simulink model "DpfIntfc_Delivery"  (Simulink 8.2)
settings: Solver=FixedStepDiscrete  StartTime=0.0  StopTime=10.0  FixedStep=0.001  RelTol=1e-3
undefined symbols (not defined in the file): DiscIntNeverNeededParam
libraries: simulink x15, DpfIntfc_Lib x1
(part 1 of 2)
settings Model: Creator=u13x50  LastModifiedBy=u13x50
settings DataIOCC: LimitDataPoints=off  SignalLoggingSaveFormat=Dataset  SaveOutput=off  SaveTime=off
settings OptimizationCC: InlineParams=on  ZeroExternalMemoryAtStartup=off  ZeroInternalMemoryAtStartup=off  InitFltsAndDblsToZero=on  EfficientMapNaN2IntZero=off  OptimizeModelRefInitCode=on  LifeSpan=Inf
settings DebuggingCC: SignalInfNanChecking=error  SignalRangeChecking=error  ReadBeforeWriteMsg=DisableAll  WriteAfterWriteMsg=DisableAll  WriteAfterReadMsg=DisableAll  InheritedTsInSrcMsg=none  UnderSpecifiedDataTypeMsg=error
settings ModelReferenceCC: ModelReferenceNumInstancesAllowed=Single
settings RTWCC: SystemTargetFile=ert.tlc  GenCodeOnly=on  GenerateMakefile=off  TemplateMakefile=ert_default_tmf  Description=Embedded Coder  GenerateReport=on  ProcessScript=ert_make_rtw_hook  IncludeHyperlinkInReport=on  LaunchReport=on
settings CodeAppCC: IgnoreCustomStorageClasses=off  CustomSymbolStrType=$N$R$M  SimulinkBlockComments=off  InternalIdentifier=Classic
settings ERTTargetCC: CodeReplacementLibrary=ANSI_C  UtilityFuncGeneration=Shared location  MultiwordLength=2048  IncludeMdlTerminateFcn=off  SuppressErrorStatus=on  SupportNonFinite=off  SupportComplex=off  ParenthesesLevel=Maximum  InlinedParameterPlacement=NonHierarchical  ERTCustomFileTemplate=example_file_process.tlc  ConvertIfToSwitch=off  SuppressUnreachableDefaultCases=off

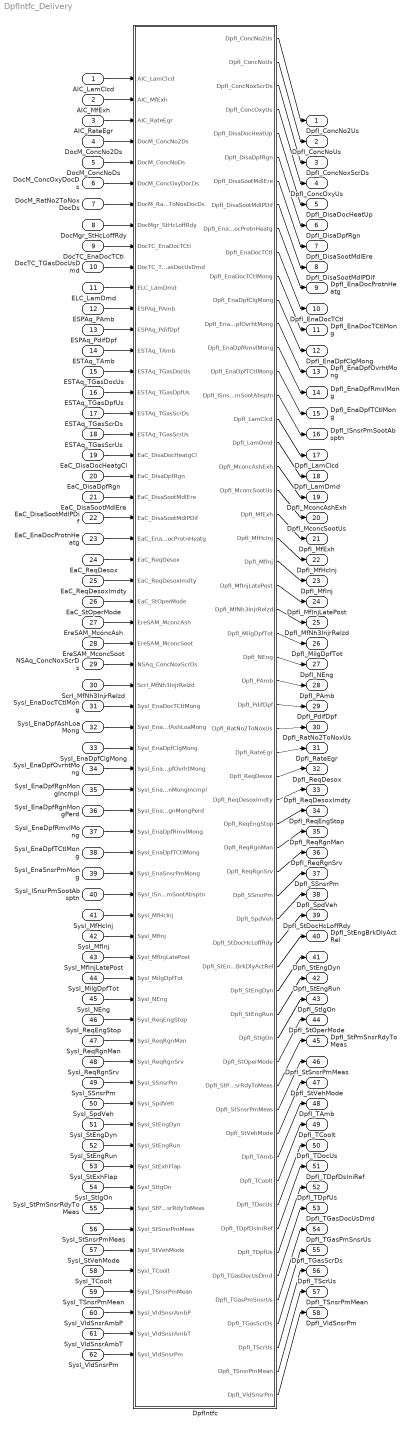
== system DpfIntfc_Delivery ==
  AIC_LamClcd : Inport
  AIC_MfExh : Inport  Port=2
  AIC_RateEgr : Inport  Port=3
  DocM_ConcNo2Ds : Inport  Port=4
  DocM_ConcNoDs : Inport  Port=5
  DocM_ConcOxyDocDs : Inport  Port=6
  DocM_RatNo2ToNoxDocDs : Inport  Port=7
  DocMgr_StHcLoffRdy : Inport  Port=8
  DocTC_EnaDocTCtl : Inport  Port=9
  DocTC_TGasDocUsDmd : Inport  Port=10
  ELC_LamDmd : Inport  Port=11
  ESPAq_PAmb : Inport  Port=12
  ESPAq_PdifDpf : Inport  Port=13
  ESTAq_TAmb : Inport  Port=14
  ESTAq_TGasDocUs : Inport  Port=15
  ESTAq_TGasDpfUs : Inport  Port=16
  ESTAq_TGasScrDs : Inport  Port=17
  ESTAq_TGasScrUs : Inport  Port=18
  EaC_DisaDocHeatgCl : Inport  Port=19
  EaC_DisaDpfRgn : Inport  Port=20
  EaC_DisaSootMdlEre : Inport  Port=21
  EaC_DisaSootMdlPDif : Inport  Port=22
  EaC_EnaDocProtnHeatg : Inport  Port=23
  EaC_ReqDesox : Inport  Port=24
  EaC_ReqDesoxImdty : Inport  Port=25
  EaC_StOperMode : Inport  Port=26
  EreSAM_MconcAsh : Inport  Port=27
  EreSAM_MconcSoot : Inport  Port=28
  NSAq_ConcNoxScrDs : Inport  Port=29
  ScrI_MfNh3InjrRelzd : Inport  Port=30
  SysI_EnaDocTCtlMong : Inport  Port=31
  SysI_EnaDpfAshLoaMong : Inport  Port=32
  SysI_EnaDpfClgMong : Inport  Port=33
  SysI_EnaDpfOvrhtMong : Inport  Port=34
  SysI_EnaDpfRgnMongIncmpl : Inport  Port=35
  SysI_EnaDpfRgnMongPerd : Inport  Port=36
  SysI_EnaDpfRmvlMong : Inport  Port=37
  SysI_EnaDpfTCtlMong : Inport  Port=38
  SysI_EnaSnsrPmMong : Inport  Port=39
  SysI_ISnsrPmSootAbsptn : Inport  Port=40
  SysI_MfHcInj : Inport  Port=41
  SysI_MfInj : Inport  Port=42
  SysI_MfInjLatePost : Inport  Port=43
  SysI_MilgDpfTot : Inport  Port=44
  SysI_NEng : Inport  Port=45
  SysI_ReqEngStop : Inport  Port=46
  SysI_ReqRgnMan : Inport  Port=47
  SysI_ReqRgnSrv : Inport  Port=48
  SysI_SSnsrPm : Inport  Port=49
  SysI_SpdVeh : Inport  Port=50
  SysI_StEngDyn : Inport  Port=51
  SysI_StEngRun : Inport  Port=52
  SysI_StExhFlap : Inport  Port=53
  SysI_StIgOn : Inport  Port=54
  SysI_StPmSnsrRdyToMeas : Inport  Port=55
  SysI_StSnsrPmMeas : Inport  Port=56
  SysI_StVehMode : Inport  Port=57
  SysI_TCoolt : Inport  Port=58
  SysI_TSnsrPmMean : Inport  Port=59
  SysI_VldSnsrAmbP : Inport  Port=60
  SysI_VldSnsrAmbT : Inport  Port=61
  SysI_VldSnsrPm : Inport  Port=62
  DpfIntfc : Subsystem
  DpfI_ConcNo2Us : Outport
  DpfI_ConcNoUs : Outport  Port=2
  DpfI_ConcNoxScrDs : Outport  Port=3
  DpfI_ConcOxyUs : Outport  Port=4
  DpfI_DisaDocHeatUp : Outport  Port=5
  DpfI_DisaDpfRgn : Outport  Port=6
  DpfI_DisaSootMdlEre : Outport  Port=7
  DpfI_DisaSootMdlPDif : Outport  Port=8
  DpfI_EnaDocProtnHeatg : Outport  Port=9
  DpfI_EnaDocTCtl : Outport  Port=10
  DpfI_EnaDocTCtlMong : Outport  Port=11
  DpfI_EnaDpfClgMong : Outport  Port=12
  DpfI_EnaDpfOvrhtMong : Outport  Port=13
  DpfI_EnaDpfRmvlMong : Outport  Port=14
  DpfI_EnaDpfTCtlMong : Outport  Port=15
  DpfI_ISnsrPmSootAbsptn : Outport  Port=16
  DpfI_LamClcd : Outport  Port=17
  DpfI_LamDmd : Outport  Port=18
  DpfI_MconcAshExh : Outport  Port=19
  DpfI_MconcSootUs : Outport  Port=20
  DpfI_MfExh : Outport  Port=21
  DpfI_MfHcInj : Outport  Port=22
  DpfI_MfInj : Outport  Port=23
  DpfI_MfInjLatePost : Outport  Port=24
  DpfI_MfNh3InjrRelzd : Outport  Port=25
  DpfI_MilgDpfTot : Outport  Port=26
  DpfI_NEng : Outport  Port=27
  DpfI_PAmb : Outport  Port=28
  DpfI_PdifDpf : Outport  Port=29
  DpfI_RatNo2ToNoxUs : Outport  Port=30
  DpfI_RateEgr : Outport  Port=31
  DpfI_ReqDesox : Outport  Port=32
  DpfI_ReqDesoxImdty : Outport  Port=33
  DpfI_ReqEngStop : Outport  Port=34
  DpfI_ReqRgnMan : Outport  Port=35
  DpfI_ReqRgnSrv : Outport  Port=36
  DpfI_SSnsrPm : Outport  Port=37
  DpfI_SpdVeh : Outport  Port=38
  DpfI_StDocHcLoffRdy : Outport  Port=39
  DpfI_StEngBrkDlyActRel : Outport  Port=40
  DpfI_StEngDyn : Outport  Port=41
  DpfI_StEngRun : Outport  Port=42
  DpfI_StIgOn : Outport  Port=43
  DpfI_StOperMode : Outport  Port=44
  DpfI_StPmSnsrRdyToMeas : Outport  Port=45
  DpfI_StSnsrPmMeas : Outport  Port=46
  DpfI_StVehMode : Outport  Port=47
  DpfI_TAmb : Outport  Port=48
  DpfI_TCoolt : Outport  Port=49
  DpfI_TDocUs : Outport  Port=50
  DpfI_TDpfDsIniRef : Outport  Port=51
  DpfI_TDpfUs : Outport  Port=52
  DpfI_TGasDocUsDmd : Outport  Port=53
  DpfI_TGasPmSnsrUs : Outport  Port=54
  DpfI_TGasScrDs : Outport  Port=55
  DpfI_TScrUs : Outport  Port=56
  DpfI_TSnsrPmMean : Outport  Port=57
  DpfI_VldSnsrPm : Outport  Port=58
  wires:
  AIC_LamClcd/1 -> DpfIntfc/1(AIC_LamClcd)
  AIC_MfExh/1 -> DpfIntfc/2(AIC_MfExh)
  AIC_RateEgr/1 -> DpfIntfc/3(AIC_RateEgr)
  DocM_ConcNo2Ds/1 -> DpfIntfc/4(DocM_ConcNo2Ds)
  DocM_ConcNoDs/1 -> DpfIntfc/5(DocM_ConcNoDs)
  DocM_ConcOxyDocDs/1 -> DpfIntfc/6(DocM_ConcOxyDocDs)
  DocM_RatNo2ToNoxDocDs/1 -> DpfIntfc/7(DocM_RatNo2ToNoxDocDs)
  DocMgr_StHcLoffRdy/1 -> DpfIntfc/8(DocMgr_StHcLoffRdy)
  DocTC_EnaDocTCtl/1 -> DpfIntfc/9(DocTC_EnaDocTCtl)
  DocTC_TGasDocUsDmd/1 -> DpfIntfc/10(DocTC_TGasDocUsDmd)
  ELC_LamDmd/1 -> DpfIntfc/11(ELC_LamDmd)
  ESPAq_PAmb/1 -> DpfIntfc/12(ESPAq_PAmb)
  ESPAq_PdifDpf/1 -> DpfIntfc/13(ESPAq_PdifDpf)
  ESTAq_TAmb/1 -> DpfIntfc/14(ESTAq_TAmb)
  ESTAq_TGasDocUs/1 -> DpfIntfc/15(ESTAq_TGasDocUs)
  ESTAq_TGasDpfUs/1 -> DpfIntfc/16(ESTAq_TGasDpfUs)
  ESTAq_TGasScrDs/1 -> DpfIntfc/17(ESTAq_TGasScrDs)
  ESTAq_TGasScrUs/1 -> DpfIntfc/18(ESTAq_TGasScrUs)
  EaC_DisaDocHeatgCl/1 -> DpfIntfc/19(EaC_DisaDocHeatgCl)
  EaC_DisaDpfRgn/1 -> DpfIntfc/20(EaC_DisaDpfRgn)
  EaC_DisaSootMdlEre/1 -> DpfIntfc/21(EaC_DisaSootMdlEre)
  EaC_DisaSootMdlPDif/1 -> DpfIntfc/22(EaC_DisaSootMdlPDif)
  EaC_EnaDocProtnHeatg/1 -> DpfIntfc/23(EaC_EnaDocProtnHeatg)
  EaC_ReqDesox/1 -> DpfIntfc/24(EaC_ReqDesox)
  EaC_ReqDesoxImdty/1 -> DpfIntfc/25(EaC_ReqDesoxImdty)
  EaC_StOperMode/1 -> DpfIntfc/26(EaC_StOperMode)
  EreSAM_MconcAsh/1 -> DpfIntfc/27(EreSAM_MconcAsh)
  EreSAM_MconcSoot/1 -> DpfIntfc/28(EreSAM_MconcSoot)
  NSAq_ConcNoxScrDs/1 -> DpfIntfc/29(NSAq_ConcNoxScrDs)
  ScrI_MfNh3InjrRelzd/1 -> DpfIntfc/30(ScrI_MfNh3InjrRelzd)
  SysI_EnaDocTCtlMong/1 -> DpfIntfc/31(SysI_EnaDocTCtlMong)
  SysI_EnaDpfAshLoaMong/1 -> DpfIntfc/32(SysI_EnaDpfAshLoaMong)
  SysI_EnaDpfClgMong/1 -> DpfIntfc/33(SysI_EnaDpfClgMong)
  SysI_EnaDpfOvrhtMong/1 -> DpfIntfc/34(SysI_EnaDpfOvrhtMong)
  SysI_EnaDpfRgnMongIncmpl/1 -> DpfIntfc/35(SysI_EnaDpfRgnMongIncmpl)
  SysI_EnaDpfRgnMongPerd/1 -> DpfIntfc/36(SysI_EnaDpfRgnMongPerd)
  SysI_EnaDpfRmvlMong/1 -> DpfIntfc/37(SysI_EnaDpfRmvlMong)
  SysI_EnaDpfTCtlMong/1 -> DpfIntfc/38(SysI_EnaDpfTCtlMong)
  SysI_EnaSnsrPmMong/1 -> DpfIntfc/39(SysI_EnaSnsrPmMong)
  SysI_ISnsrPmSootAbsptn/1 -> DpfIntfc/40(SysI_ISnsrPmSootAbsptn)
  SysI_MfHcInj/1 -> DpfIntfc/41(SysI_MfHcInj)
  SysI_MfInj/1 -> DpfIntfc/42(SysI_MfInj)
  SysI_MfInjLatePost/1 -> DpfIntfc/43(SysI_MfInjLatePost)
  SysI_MilgDpfTot/1 -> DpfIntfc/44(SysI_MilgDpfTot)
  SysI_NEng/1 -> DpfIntfc/45(SysI_NEng)
  SysI_ReqEngStop/1 -> DpfIntfc/46(SysI_ReqEngStop)
  SysI_ReqRgnMan/1 -> DpfIntfc/47(SysI_ReqRgnMan)
  SysI_ReqRgnSrv/1 -> DpfIntfc/48(SysI_ReqRgnSrv)
  SysI_SSnsrPm/1 -> DpfIntfc/49(SysI_SSnsrPm)
  SysI_SpdVeh/1 -> DpfIntfc/50(SysI_SpdVeh)
  SysI_StEngDyn/1 -> DpfIntfc/51(SysI_StEngDyn)
  SysI_StEngRun/1 -> DpfIntfc/52(SysI_StEngRun)
  SysI_StExhFlap/1 -> DpfIntfc/53(SysI_StExhFlap)
  SysI_StIgOn/1 -> DpfIntfc/54(SysI_StIgOn)
  SysI_StPmSnsrRdyToMeas/1 -> DpfIntfc/55(SysI_StPmSnsrRdyToMeas)
  SysI_StSnsrPmMeas/1 -> DpfIntfc/56(SysI_StSnsrPmMeas)
  SysI_StVehMode/1 -> DpfIntfc/57(SysI_StVehMode)
  SysI_TCoolt/1 -> DpfIntfc/58(SysI_TCoolt)
  SysI_TSnsrPmMean/1 -> DpfIntfc/59(SysI_TSnsrPmMean)
  SysI_VldSnsrAmbP/1 -> DpfIntfc/60(SysI_VldSnsrAmbP)
  SysI_VldSnsrAmbT/1 -> DpfIntfc/61(SysI_VldSnsrAmbT)
  SysI_VldSnsrPm/1 -> DpfIntfc/62(SysI_VldSnsrPm)
  DpfIntfc/1(DpfI_ConcNo2Us) -> DpfI_ConcNo2Us/1
  DpfIntfc/2(DpfI_ConcNoUs) -> DpfI_ConcNoUs/1
  DpfIntfc/3(DpfI_ConcNoxScrDs) -> DpfI_ConcNoxScrDs/1
  DpfIntfc/4(DpfI_ConcOxyUs) -> DpfI_ConcOxyUs/1
  DpfIntfc/5(DpfI_DisaDocHeatUp) -> DpfI_DisaDocHeatUp/1
  DpfIntfc/6(DpfI_DisaDpfRgn) -> DpfI_DisaDpfRgn/1
  DpfIntfc/7(DpfI_DisaSootMdlEre) -> DpfI_DisaSootMdlEre/1
  DpfIntfc/8(DpfI_DisaSootMdlPDif) -> DpfI_DisaSootMdlPDif/1
  DpfIntfc/9(DpfI_EnaDocProtnHeatg) -> DpfI_EnaDocProtnHeatg/1
  DpfIntfc/10(DpfI_EnaDocTCtl) -> DpfI_EnaDocTCtl/1
  DpfIntfc/11(DpfI_EnaDocTCtlMong) -> DpfI_EnaDocTCtlMong/1
  DpfIntfc/12(DpfI_EnaDpfClgMong) -> DpfI_EnaDpfClgMong/1
  DpfIntfc/13(DpfI_EnaDpfOvrhtMong) -> DpfI_EnaDpfOvrhtMong/1
  DpfIntfc/14(DpfI_EnaDpfRmvlMong) -> DpfI_EnaDpfRmvlMong/1
  DpfIntfc/15(DpfI_EnaDpfTCtlMong) -> DpfI_EnaDpfTCtlMong/1
  DpfIntfc/16(DpfI_ISnsrPmSootAbsptn) -> DpfI_ISnsrPmSootAbsptn/1
  DpfIntfc/17(DpfI_LamClcd) -> DpfI_LamClcd/1
  DpfIntfc/18(DpfI_LamDmd) -> DpfI_LamDmd/1
  DpfIntfc/19(DpfI_MconcAshExh) -> DpfI_MconcAshExh/1
  DpfIntfc/20(DpfI_MconcSootUs) -> DpfI_MconcSootUs/1
  DpfIntfc/21(DpfI_MfExh) -> DpfI_MfExh/1
  DpfIntfc/22(DpfI_MfHcInj) -> DpfI_MfHcInj/1
  DpfIntfc/23(DpfI_MfInj) -> DpfI_MfInj/1
  DpfIntfc/24(DpfI_MfInjLatePost) -> DpfI_MfInjLatePost/1
  DpfIntfc/25(DpfI_MfNh3InjrRelzd) -> DpfI_MfNh3InjrRelzd/1
  DpfIntfc/26(DpfI_MilgDpfTot) -> DpfI_MilgDpfTot/1
  DpfIntfc/27(DpfI_NEng) -> DpfI_NEng/1
  DpfIntfc/28(DpfI_PAmb) -> DpfI_PAmb/1
  DpfIntfc/29(DpfI_PdifDpf) -> DpfI_PdifDpf/1
  DpfIntfc/30(DpfI_RatNo2ToNoxUs) -> DpfI_RatNo2ToNoxUs/1
  DpfIntfc/31(DpfI_RateEgr) -> DpfI_RateEgr/1
  DpfIntfc/32(DpfI_ReqDesox) -> DpfI_ReqDesox/1
  DpfIntfc/33(DpfI_ReqDesoxImdty) -> DpfI_ReqDesoxImdty/1
  DpfIntfc/34(DpfI_ReqEngStop) -> DpfI_ReqEngStop/1
  DpfIntfc/35(DpfI_ReqRgnMan) -> DpfI_ReqRgnMan/1
  DpfIntfc/36(DpfI_ReqRgnSrv) -> DpfI_ReqRgnSrv/1
  DpfIntfc/37(DpfI_SSnsrPm) -> DpfI_SSnsrPm/1
  DpfIntfc/38(DpfI_SpdVeh) -> DpfI_SpdVeh/1
  DpfIntfc/39(DpfI_StDocHcLoffRdy) -> DpfI_StDocHcLoffRdy/1
  DpfIntfc/40(DpfI_StEngBrkDlyActRel) -> DpfI_StEngBrkDlyActRel/1
  DpfIntfc/41(DpfI_StEngDyn) -> DpfI_StEngDyn/1
  DpfIntfc/42(DpfI_StEngRun) -> DpfI_StEngRun/1
  DpfIntfc/43(DpfI_StIgOn) -> DpfI_StIgOn/1
  DpfIntfc/44(DpfI_StOperMode) -> DpfI_StOperMode/1
  DpfIntfc/45(DpfI_StPmSnsrRdyToMeas) -> DpfI_StPmSnsrRdyToMeas/1
  DpfIntfc/46(DpfI_StSnsrPmMeas) -> DpfI_StSnsrPmMeas/1
  DpfIntfc/47(DpfI_StVehMode) -> DpfI_StVehMode/1
  DpfIntfc/48(DpfI_TAmb) -> DpfI_TAmb/1
  DpfIntfc/49(DpfI_TCoolt) -> DpfI_TCoolt/1
  DpfIntfc/50(DpfI_TDocUs) -> DpfI_TDocUs/1
  DpfIntfc/51(DpfI_TDpfDsIniRef) -> DpfI_TDpfDsIniRef/1
  DpfIntfc/52(DpfI_TDpfUs) -> DpfI_TDpfUs/1
  DpfIntfc/53(DpfI_TGasDocUsDmd) -> DpfI_TGasDocUsDmd/1
  DpfIntfc/54(DpfI_TGasPmSnsrUs) -> DpfI_TGasPmSnsrUs/1
  DpfIntfc/55(DpfI_TGasScrDs) -> DpfI_TGasScrDs/1
  DpfIntfc/56(DpfI_TScrUs) -> DpfI_TScrUs/1
  DpfIntfc/57(DpfI_TSnsrPmMean) -> DpfI_TSnsrPmMean/1
  DpfIntfc/58(DpfI_VldSnsrPm) -> DpfI_VldSnsrPm/1

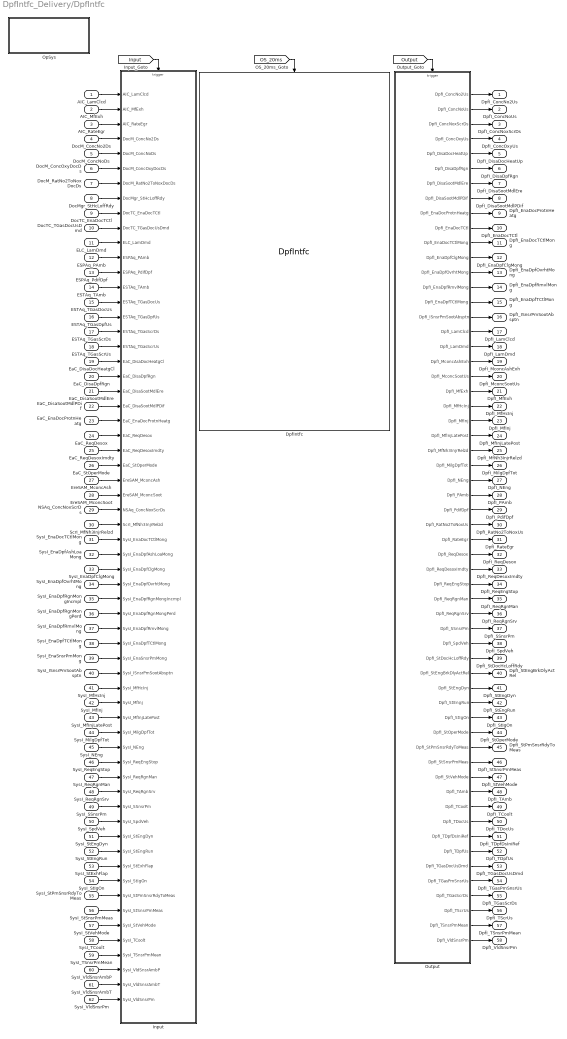
== system DpfIntfc_Delivery/DpfIntfc ==
  AIC_LamClcd : Inport
  AIC_MfExh : Inport  Port=2
  AIC_RateEgr : Inport  Port=3
  DocM_ConcNo2Ds : Inport  Port=4
  DocM_ConcNoDs : Inport  Port=5
  DocM_ConcOxyDocDs : Inport  Port=6
  DocM_RatNo2ToNoxDocDs : Inport  Port=7
  DocMgr_StHcLoffRdy : Inport  Port=8
  DocTC_EnaDocTCtl : Inport  Port=9
  DocTC_TGasDocUsDmd : Inport  Port=10
  ELC_LamDmd : Inport  Port=11
  ESPAq_PAmb : Inport  Port=12
  ESPAq_PdifDpf : Inport  Port=13
  ESTAq_TAmb : Inport  Port=14
  ESTAq_TGasDocUs : Inport  Port=15
  ESTAq_TGasDpfUs : Inport  Port=16
  ESTAq_TGasScrDs : Inport  Port=17
  ESTAq_TGasScrUs : Inport  Port=18
  EaC_DisaDocHeatgCl : Inport  Port=19
  EaC_DisaDpfRgn : Inport  Port=20
  EaC_DisaSootMdlEre : Inport  Port=21
  EaC_DisaSootMdlPDif : Inport  Port=22
  EaC_EnaDocProtnHeatg : Inport  Port=23
  EaC_ReqDesox : Inport  Port=24
  EaC_ReqDesoxImdty : Inport  Port=25
  EaC_StOperMode : Inport  Port=26
  EreSAM_MconcAsh : Inport  Port=27
  EreSAM_MconcSoot : Inport  Port=28
  NSAq_ConcNoxScrDs : Inport  Port=29
  ScrI_MfNh3InjrRelzd : Inport  Port=30
  SysI_EnaDocTCtlMong : Inport  Port=31
  SysI_EnaDpfAshLoaMong : Inport  Port=32
  SysI_EnaDpfClgMong : Inport  Port=33
  SysI_EnaDpfOvrhtMong : Inport  Port=34
  SysI_EnaDpfRgnMongIncmpl : Inport  Port=35
  SysI_EnaDpfRgnMongPerd : Inport  Port=36
  SysI_EnaDpfRmvlMong : Inport  Port=37
  SysI_EnaDpfTCtlMong : Inport  Port=38
  SysI_EnaSnsrPmMong : Inport  Port=39
  SysI_ISnsrPmSootAbsptn : Inport  Port=40
  SysI_MfHcInj : Inport  Port=41
  SysI_MfInj : Inport  Port=42
  SysI_MfInjLatePost : Inport  Port=43
  SysI_MilgDpfTot : Inport  Port=44
  SysI_NEng : Inport  Port=45
  SysI_ReqEngStop : Inport  Port=46
  SysI_ReqRgnMan : Inport  Port=47
  SysI_ReqRgnSrv : Inport  Port=48
  SysI_SSnsrPm : Inport  Port=49
  SysI_SpdVeh : Inport  Port=50
  SysI_StEngDyn : Inport  Port=51
  SysI_StEngRun : Inport  Port=52
  SysI_StExhFlap : Inport  Port=53
  SysI_StIgOn : Inport  Port=54
  SysI_StPmSnsrRdyToMeas : Inport  Port=55
  SysI_StSnsrPmMeas : Inport  Port=56
  SysI_StVehMode : Inport  Port=57
  SysI_TCoolt : Inport  Port=58
  SysI_TSnsrPmMean : Inport  Port=59
  SysI_VldSnsrAmbP : Inport  Port=60
  SysI_VldSnsrAmbT : Inport  Port=61
  SysI_VldSnsrPm : Inport  Port=62
  DpfIntfc : DpfIntfc_Lib/DpfIntfc  SystemSampleTime=-1
  Input : Subsystem  TreatAsAtomicUnit=on
  OpSys : Subsystem
      mask Display: disp('Operating System')
  Output : Subsystem  TreatAsAtomicUnit=on
  DpfI_ConcNo2Us : Outport
  DpfI_ConcNoUs : Outport  Port=2
  DpfI_ConcNoxScrDs : Outport  Port=3
  DpfI_ConcOxyUs : Outport  Port=4
  DpfI_DisaDocHeatUp : Outport  Port=5
  DpfI_DisaDpfRgn : Outport  Port=6
  DpfI_DisaSootMdlEre : Outport  Port=7
  DpfI_DisaSootMdlPDif : Outport  Port=8
  DpfI_EnaDocProtnHeatg : Outport  Port=9
  DpfI_EnaDocTCtl : Outport  Port=10
  DpfI_EnaDocTCtlMong : Outport  Port=11
  DpfI_EnaDpfClgMong : Outport  Port=12
  DpfI_EnaDpfOvrhtMong : Outport  Port=13
  DpfI_EnaDpfRmvlMong : Outport  Port=14
  DpfI_EnaDpfTCtlMong : Outport  Port=15
  DpfI_ISnsrPmSootAbsptn : Outport  Port=16
  DpfI_LamClcd : Outport  Port=17
  DpfI_LamDmd : Outport  Port=18
  DpfI_MconcAshExh : Outport  Port=19
  DpfI_MconcSootUs : Outport  Port=20
  DpfI_MfExh : Outport  Port=21
  DpfI_MfHcInj : Outport  Port=22
  DpfI_MfInj : Outport  Port=23
  DpfI_MfInjLatePost : Outport  Port=24
  DpfI_MfNh3InjrRelzd : Outport  Port=25
  DpfI_MilgDpfTot : Outport  Port=26
  DpfI_NEng : Outport  Port=27
  DpfI_PAmb : Outport  Port=28
  DpfI_PdifDpf : Outport  Port=29
  DpfI_RatNo2ToNoxUs : Outport  Port=30
  DpfI_RateEgr : Outport  Port=31
  DpfI_ReqDesox : Outport  Port=32
  DpfI_ReqDesoxImdty : Outport  Port=33
  DpfI_ReqEngStop : Outport  Port=34
  DpfI_ReqRgnMan : Outport  Port=35
  DpfI_ReqRgnSrv : Outport  Port=36
  DpfI_SSnsrPm : Outport  Port=37
  DpfI_SpdVeh : Outport  Port=38
  DpfI_StDocHcLoffRdy : Outport  Port=39
  DpfI_StEngBrkDlyActRel : Outport  Port=40
  DpfI_StEngDyn : Outport  Port=41
  DpfI_StEngRun : Outport  Port=42
  DpfI_StIgOn : Outport  Port=43
  DpfI_StOperMode : Outport  Port=44
  DpfI_StPmSnsrRdyToMeas : Outport  Port=45
  DpfI_StSnsrPmMeas : Outport  Port=46
  DpfI_StVehMode : Outport  Port=47
  DpfI_TAmb : Outport  Port=48
  DpfI_TCoolt : Outport  Port=49
  DpfI_TDocUs : Outport  Port=50
  DpfI_TDpfDsIniRef : Outport  Port=51
  DpfI_TDpfUs : Outport  Port=52
  DpfI_TGasDocUsDmd : Outport  Port=53
  DpfI_TGasPmSnsrUs : Outport  Port=54
  DpfI_TGasScrDs : Outport  Port=55
  DpfI_TScrUs : Outport  Port=56
  DpfI_TSnsrPmMean : Outport  Port=57
  DpfI_VldSnsrPm : Outport  Port=58
  wires:
  AIC_LamClcd/1 -> Input/1(AIC_LamClcd)
  AIC_MfExh/1 -> Input/2(AIC_MfExh)
  AIC_RateEgr/1 -> Input/3(AIC_RateEgr)
  DocM_ConcNo2Ds/1 -> Input/4(DocM_ConcNo2Ds)
  DocM_ConcNoDs/1 -> Input/5(DocM_ConcNoDs)
  DocM_ConcOxyDocDs/1 -> Input/6(DocM_ConcOxyDocDs)
  DocM_RatNo2ToNoxDocDs/1 -> Input/7(DocM_RatNo2ToNoxDocDs)
  DocMgr_StHcLoffRdy/1 -> Input/8(DocMgr_StHcLoffRdy)
  DocTC_EnaDocTCtl/1 -> Input/9(DocTC_EnaDocTCtl)
  DocTC_TGasDocUsDmd/1 -> Input/10(DocTC_TGasDocUsDmd)
  ELC_LamDmd/1 -> Input/11(ELC_LamDmd)
  ESPAq_PAmb/1 -> Input/12(ESPAq_PAmb)
  ESPAq_PdifDpf/1 -> Input/13(ESPAq_PdifDpf)
  ESTAq_TAmb/1 -> Input/14(ESTAq_TAmb)
  ESTAq_TGasDocUs/1 -> Input/15(ESTAq_TGasDocUs)
  ESTAq_TGasDpfUs/1 -> Input/16(ESTAq_TGasDpfUs)
  ESTAq_TGasScrDs/1 -> Input/17(ESTAq_TGasScrDs)
  ESTAq_TGasScrUs/1 -> Input/18(ESTAq_TGasScrUs)
  EaC_DisaDocHeatgCl/1 -> Input/19(EaC_DisaDocHeatgCl)
  EaC_DisaDpfRgn/1 -> Input/20(EaC_DisaDpfRgn)
  EaC_DisaSootMdlEre/1 -> Input/21(EaC_DisaSootMdlEre)
  EaC_DisaSootMdlPDif/1 -> Input/22(EaC_DisaSootMdlPDif)
  EaC_EnaDocProtnHeatg/1 -> Input/23(EaC_EnaDocProtnHeatg)
  EaC_ReqDesox/1 -> Input/24(EaC_ReqDesox)
  EaC_ReqDesoxImdty/1 -> Input/25(EaC_ReqDesoxImdty)
  EaC_StOperMode/1 -> Input/26(EaC_StOperMode)
  EreSAM_MconcAsh/1 -> Input/27(EreSAM_MconcAsh)
  EreSAM_MconcSoot/1 -> Input/28(EreSAM_MconcSoot)
  NSAq_ConcNoxScrDs/1 -> Input/29(NSAq_ConcNoxScrDs)
  ScrI_MfNh3InjrRelzd/1 -> Input/30(ScrI_MfNh3InjrRelzd)
  SysI_EnaDocTCtlMong/1 -> Input/31(SysI_EnaDocTCtlMong)
  SysI_EnaDpfAshLoaMong/1 -> Input/32(SysI_EnaDpfAshLoaMong)
  SysI_EnaDpfClgMong/1 -> Input/33(SysI_EnaDpfClgMong)
  SysI_EnaDpfOvrhtMong/1 -> Input/34(SysI_EnaDpfOvrhtMong)
  SysI_EnaDpfRgnMongIncmpl/1 -> Input/35(SysI_EnaDpfRgnMongIncmpl)
  SysI_EnaDpfRgnMongPerd/1 -> Input/36(SysI_EnaDpfRgnMongPerd)
  SysI_EnaDpfRmvlMong/1 -> Input/37(SysI_EnaDpfRmvlMong)
  SysI_EnaDpfTCtlMong/1 -> Input/38(SysI_EnaDpfTCtlMong)
  SysI_EnaSnsrPmMong/1 -> Input/39(SysI_EnaSnsrPmMong)
  SysI_ISnsrPmSootAbsptn/1 -> Input/40(SysI_ISnsrPmSootAbsptn)
  SysI_MfHcInj/1 -> Input/41(SysI_MfHcInj)
  SysI_MfInj/1 -> Input/42(SysI_MfInj)
  SysI_MfInjLatePost/1 -> Input/43(SysI_MfInjLatePost)
  SysI_MilgDpfTot/1 -> Input/44(SysI_MilgDpfTot)
  SysI_NEng/1 -> Input/45(SysI_NEng)
  SysI_ReqEngStop/1 -> Input/46(SysI_ReqEngStop)
  SysI_ReqRgnMan/1 -> Input/47(SysI_ReqRgnMan)
  SysI_ReqRgnSrv/1 -> Input/48(SysI_ReqRgnSrv)
  SysI_SSnsrPm/1 -> Input/49(SysI_SSnsrPm)
  SysI_SpdVeh/1 -> Input/50(SysI_SpdVeh)
  SysI_StEngDyn/1 -> Input/51(SysI_StEngDyn)
  SysI_StEngRun/1 -> Input/52(SysI_StEngRun)
  SysI_StExhFlap/1 -> Input/53(SysI_StExhFlap)
  SysI_StIgOn/1 -> Input/54(SysI_StIgOn)
  SysI_StPmSnsrRdyToMeas/1 -> Input/55(SysI_StPmSnsrRdyToMeas)
  SysI_StSnsrPmMeas/1 -> Input/56(SysI_StSnsrPmMeas)
  SysI_StVehMode/1 -> Input/57(SysI_StVehMode)
  SysI_TCoolt/1 -> Input/58(SysI_TCoolt)
  SysI_TSnsrPmMean/1 -> Input/59(SysI_TSnsrPmMean)
  SysI_VldSnsrAmbP/1 -> Input/60(SysI_VldSnsrAmbP)
  SysI_VldSnsrAmbT/1 -> Input/61(SysI_VldSnsrAmbT)
  SysI_VldSnsrPm/1 -> Input/62(SysI_VldSnsrPm)
  Output/1(DpfI_ConcNo2Us) -> DpfI_ConcNo2Us/1
  Output/2(DpfI_ConcNoUs) -> DpfI_ConcNoUs/1
  Output/3(DpfI_ConcNoxScrDs) -> DpfI_ConcNoxScrDs/1
  Output/4(DpfI_ConcOxyUs) -> DpfI_ConcOxyUs/1
  Output/5(DpfI_DisaDocHeatUp) -> DpfI_DisaDocHeatUp/1
  Output/6(DpfI_DisaDpfRgn) -> DpfI_DisaDpfRgn/1
  Output/7(DpfI_DisaSootMdlEre) -> DpfI_DisaSootMdlEre/1
  Output/8(DpfI_DisaSootMdlPDif) -> DpfI_DisaSootMdlPDif/1
  Output/9(DpfI_EnaDocProtnHeatg) -> DpfI_EnaDocProtnHeatg/1
  Output/10(DpfI_EnaDocTCtl) -> DpfI_EnaDocTCtl/1
  Output/11(DpfI_EnaDocTCtlMong) -> DpfI_EnaDocTCtlMong/1
  Output/12(DpfI_EnaDpfClgMong) -> DpfI_EnaDpfClgMong/1
  Output/13(DpfI_EnaDpfOvrhtMong) -> DpfI_EnaDpfOvrhtMong/1
  Output/14(DpfI_EnaDpfRmvlMong) -> DpfI_EnaDpfRmvlMong/1
  Output/15(DpfI_EnaDpfTCtlMong) -> DpfI_EnaDpfTCtlMong/1
  Output/16(DpfI_ISnsrPmSootAbsptn) -> DpfI_ISnsrPmSootAbsptn/1
  Output/17(DpfI_LamClcd) -> DpfI_LamClcd/1
  Output/18(DpfI_LamDmd) -> DpfI_LamDmd/1
  Output/19(DpfI_MconcAshExh) -> DpfI_MconcAshExh/1
  Output/20(DpfI_MconcSootUs) -> DpfI_MconcSootUs/1
  Output/21(DpfI_MfExh) -> DpfI_MfExh/1
  Output/22(DpfI_MfHcInj) -> DpfI_MfHcInj/1
  Output/23(DpfI_MfInj) -> DpfI_MfInj/1
  Output/24(DpfI_MfInjLatePost) -> DpfI_MfInjLatePost/1
  Output/25(DpfI_MfNh3InjrRelzd) -> DpfI_MfNh3InjrRelzd/1
  Output/26(DpfI_MilgDpfTot) -> DpfI_MilgDpfTot/1
  Output/27(DpfI_NEng) -> DpfI_NEng/1
  Output/28(DpfI_PAmb) -> DpfI_PAmb/1
  Output/29(DpfI_PdifDpf) -> DpfI_PdifDpf/1
  Output/30(DpfI_RatNo2ToNoxUs) -> DpfI_RatNo2ToNoxUs/1
  Output/31(DpfI_RateEgr) -> DpfI_RateEgr/1
  Output/32(DpfI_ReqDesox) -> DpfI_ReqDesox/1
  Output/33(DpfI_ReqDesoxImdty) -> DpfI_ReqDesoxImdty/1
  Output/34(DpfI_ReqEngStop) -> DpfI_ReqEngStop/1
  Output/35(DpfI_ReqRgnMan) -> DpfI_ReqRgnMan/1
  Output/36(DpfI_ReqRgnSrv) -> DpfI_ReqRgnSrv/1
  Output/37(DpfI_SSnsrPm) -> DpfI_SSnsrPm/1
  Output/38(DpfI_SpdVeh) -> DpfI_SpdVeh/1
  Output/39(DpfI_StDocHcLoffRdy) -> DpfI_StDocHcLoffRdy/1
  Output/40(DpfI_StEngBrkDlyActRel) -> DpfI_StEngBrkDlyActRel/1
  Output/41(DpfI_StEngDyn) -> DpfI_StEngDyn/1
  Output/42(DpfI_StEngRun) -> DpfI_StEngRun/1
  Output/43(DpfI_StIgOn) -> DpfI_StIgOn/1
  Output/44(DpfI_StOperMode) -> DpfI_StOperMode/1
  Output/45(DpfI_StPmSnsrRdyToMeas) -> DpfI_StPmSnsrRdyToMeas/1
  Output/46(DpfI_StSnsrPmMeas) -> DpfI_StSnsrPmMeas/1
  Output/47(DpfI_StVehMode) -> DpfI_StVehMode/1
  Output/48(DpfI_TAmb) -> DpfI_TAmb/1
  Output/49(DpfI_TCoolt) -> DpfI_TCoolt/1
  Output/50(DpfI_TDocUs) -> DpfI_TDocUs/1
  Output/51(DpfI_TDpfDsIniRef) -> DpfI_TDpfDsIniRef/1
  Output/52(DpfI_TDpfUs) -> DpfI_TDpfUs/1
  Output/53(DpfI_TGasDocUsDmd) -> DpfI_TGasDocUsDmd/1
  Output/54(DpfI_TGasPmSnsrUs) -> DpfI_TGasPmSnsrUs/1
  Output/55(DpfI_TGasScrDs) -> DpfI_TGasScrDs/1
  Output/56(DpfI_TScrUs) -> DpfI_TScrUs/1
  Output/57(DpfI_TSnsrPmMean) -> DpfI_TSnsrPmMean/1
  Output/58(DpfI_VldSnsrPm) -> DpfI_VldSnsrPm/1
  [OS_20ms] -> DpfIntfc/1
  [Input] -> Input/Trigger
  [Output] -> Output/Trigger

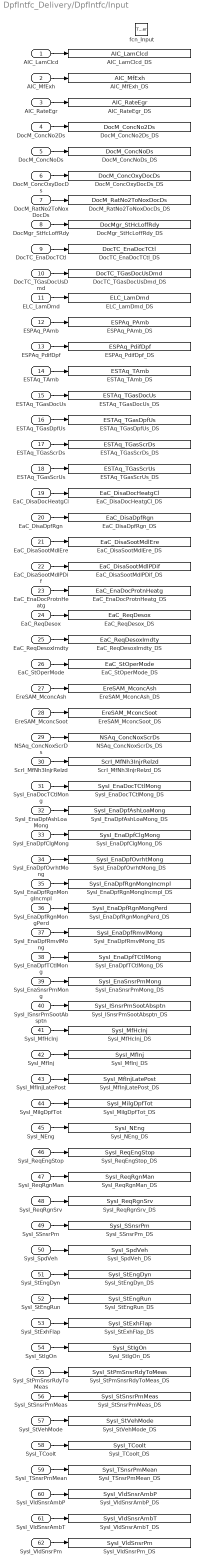
== system DpfIntfc_Delivery/DpfIntfc/Input ==
  AIC_LamClcd : Inport
  AIC_MfExh : Inport  Port=2
  AIC_RateEgr : Inport  Port=3
  DocM_ConcNo2Ds : Inport  Port=4
  DocM_ConcNoDs : Inport  Port=5
  DocM_ConcOxyDocDs : Inport  Port=6
  DocM_RatNo2ToNoxDocDs : Inport  Port=7
  DocMgr_StHcLoffRdy : Inport  Port=8
  DocTC_EnaDocTCtl : Inport  Port=9
  DocTC_TGasDocUsDmd : Inport  Port=10
  ELC_LamDmd : Inport  Port=11
  ESPAq_PAmb : Inport  Port=12
  ESPAq_PdifDpf : Inport  Port=13
  ESTAq_TAmb : Inport  Port=14
  ESTAq_TGasDocUs : Inport  Port=15
  ESTAq_TGasDpfUs : Inport  Port=16
  ESTAq_TGasScrDs : Inport  Port=17
  ESTAq_TGasScrUs : Inport  Port=18
  EaC_DisaDocHeatgCl : Inport  Port=19
  EaC_DisaDpfRgn : Inport  Port=20
  EaC_DisaSootMdlEre : Inport  Port=21
  EaC_DisaSootMdlPDif : Inport  Port=22
  EaC_EnaDocProtnHeatg : Inport  Port=23
  EaC_ReqDesox : Inport  Port=24
  EaC_ReqDesoxImdty : Inport  Port=25
  EaC_StOperMode : Inport  Port=26
  EreSAM_MconcAsh : Inport  Port=27
  EreSAM_MconcSoot : Inport  Port=28
  NSAq_ConcNoxScrDs : Inport  Port=29
  ScrI_MfNh3InjrRelzd : Inport  Port=30
  SysI_EnaDocTCtlMong : Inport  Port=31
  SysI_EnaDpfAshLoaMong : Inport  Port=32
  SysI_EnaDpfClgMong : Inport  Port=33
  SysI_EnaDpfOvrhtMong : Inport  Port=34
  SysI_EnaDpfRgnMongIncmpl : Inport  Port=35
  SysI_EnaDpfRgnMongPerd : Inport  Port=36
  SysI_EnaDpfRmvlMong : Inport  Port=37
  SysI_EnaDpfTCtlMong : Inport  Port=38
  SysI_EnaSnsrPmMong : Inport  Port=39
  SysI_ISnsrPmSootAbsptn : Inport  Port=40
  SysI_MfHcInj : Inport  Port=41
  SysI_MfInj : Inport  Port=42
  SysI_MfInjLatePost : Inport  Port=43
  SysI_MilgDpfTot : Inport  Port=44
  SysI_NEng : Inport  Port=45
  SysI_ReqEngStop : Inport  Port=46
  SysI_ReqRgnMan : Inport  Port=47
  SysI_ReqRgnSrv : Inport  Port=48
  SysI_SSnsrPm : Inport  Port=49
  SysI_SpdVeh : Inport  Port=50
  SysI_StEngDyn : Inport  Port=51
  SysI_StEngRun : Inport  Port=52
  SysI_StExhFlap : Inport  Port=53
  SysI_StIgOn : Inport  Port=54
  SysI_StPmSnsrRdyToMeas : Inport  Port=55
  SysI_StSnsrPmMeas : Inport  Port=56
  SysI_StVehMode : Inport  Port=57
  SysI_TCoolt : Inport  Port=58
  SysI_TSnsrPmMean : Inport  Port=59
  SysI_VldSnsrAmbP : Inport  Port=60
  SysI_VldSnsrAmbT : Inport  Port=61
  SysI_VldSnsrPm : Inport  Port=62
  fcn_Input : TriggerPort  TriggerType=function-call
  AIC_LamClcd_DS : DataStoreWrite  DataStoreName=AIC_LamClcd
  AIC_MfExh_DS : DataStoreWrite  DataStoreName=AIC_MfExh
  AIC_RateEgr_DS : DataStoreWrite  DataStoreName=AIC_RateEgr
  DocM_ConcNo2Ds_DS : DataStoreWrite  DataStoreName=DocM_ConcNo2Ds
  DocM_ConcNoDs_DS : DataStoreWrite  DataStoreName=DocM_ConcNoDs
  DocM_ConcOxyDocDs_DS : DataStoreWrite  DataStoreName=DocM_ConcOxyDocDs
  DocM_RatNo2ToNoxDocDs_DS : DataStoreWrite  DataStoreName=DocM_RatNo2ToNoxDocDs
  DocMgr_StHcLoffRdy_DS : DataStoreWrite  DataStoreName=DocMgr_StHcLoffRdy
  DocTC_EnaDocTCtl_DS : DataStoreWrite  DataStoreName=DocTC_EnaDocTCtl
  DocTC_TGasDocUsDmd_DS : DataStoreWrite  DataStoreName=DocTC_TGasDocUsDmd
  ELC_LamDmd_DS : DataStoreWrite  DataStoreName=ELC_LamDmd
  ESPAq_PAmb_DS : DataStoreWrite  DataStoreName=ESPAq_PAmb
  ESPAq_PdifDpf_DS : DataStoreWrite  DataStoreName=ESPAq_PdifDpf
  ESTAq_TAmb_DS : DataStoreWrite  DataStoreName=ESTAq_TAmb
  ESTAq_TGasDocUs_DS : DataStoreWrite  DataStoreName=ESTAq_TGasDocUs
  ESTAq_TGasDpfUs_DS : DataStoreWrite  DataStoreName=ESTAq_TGasDpfUs
  ESTAq_TGasScrDs_DS : DataStoreWrite  DataStoreName=ESTAq_TGasScrDs
  ESTAq_TGasScrUs_DS : DataStoreWrite  DataStoreName=ESTAq_TGasScrUs
  EaC_DisaDocHeatgCl_DS : DataStoreWrite  DataStoreName=EaC_DisaDocHeatgCl
  EaC_DisaDpfRgn_DS : DataStoreWrite  DataStoreName=EaC_DisaDpfRgn
  EaC_DisaSootMdlEre_DS : DataStoreWrite  DataStoreName=EaC_DisaSootMdlEre
  EaC_DisaSootMdlPDif_DS : DataStoreWrite  DataStoreName=EaC_DisaSootMdlPDif
  EaC_EnaDocProtnHeatg_DS : DataStoreWrite  DataStoreName=EaC_EnaDocProtnHeatg
  EaC_ReqDesoxImdty_DS : DataStoreWrite  DataStoreName=EaC_ReqDesoxImdty
  EaC_ReqDesox_DS : DataStoreWrite  DataStoreName=EaC_ReqDesox
  EaC_StOperMode_DS : DataStoreWrite  DataStoreName=EaC_StOperMode
  EreSAM_MconcAsh_DS : DataStoreWrite  DataStoreName=EreSAM_MconcAsh
  EreSAM_MconcSoot_DS : DataStoreWrite  DataStoreName=EreSAM_MconcSoot
  NSAq_ConcNoxScrDs_DS : DataStoreWrite  DataStoreName=NSAq_ConcNoxScrDs
  ScrI_MfNh3InjrRelzd_DS : DataStoreWrite  DataStoreName=ScrI_MfNh3InjrRelzd
  SysI_EnaDocTCtlMong_DS : DataStoreWrite  DataStoreName=SysI_EnaDocTCtlMong
  SysI_EnaDpfAshLoaMong_DS : DataStoreWrite  DataStoreName=SysI_EnaDpfAshLoaMong
  SysI_EnaDpfClgMong_DS : DataStoreWrite  DataStoreName=SysI_EnaDpfClgMong
  SysI_EnaDpfOvrhtMong_DS : DataStoreWrite  DataStoreName=SysI_EnaDpfOvrhtMong
  SysI_EnaDpfRgnMongIncmpl_DS : DataStoreWrite  DataStoreName=SysI_EnaDpfRgnMongIncmpl
  SysI_EnaDpfRgnMongPerd_DS : DataStoreWrite  DataStoreName=SysI_EnaDpfRgnMongPerd
  SysI_EnaDpfRmvlMong_DS : DataStoreWrite  DataStoreName=SysI_EnaDpfRmvlMong
  SysI_EnaDpfTCtlMong_DS : DataStoreWrite  DataStoreName=SysI_EnaDpfTCtlMong
  SysI_EnaSnsrPmMong_DS : DataStoreWrite  DataStoreName=SysI_EnaSnsrPmMong
  SysI_ISnsrPmSootAbsptn_DS : DataStoreWrite  DataStoreName=SysI_ISnsrPmSootAbsptn
  SysI_MfHcInj_DS : DataStoreWrite  DataStoreName=SysI_MfHcInj
  SysI_MfInjLatePost_DS : DataStoreWrite  DataStoreName=SysI_MfInjLatePost
  SysI_MfInj_DS : DataStoreWrite  DataStoreName=SysI_MfInj
  SysI_MilgDpfTot_DS : DataStoreWrite  DataStoreName=SysI_MilgDpfTot
  SysI_NEng_DS : DataStoreWrite  DataStoreName=SysI_NEng
  SysI_ReqEngStop_DS : DataStoreWrite  DataStoreName=SysI_ReqEngStop
  SysI_ReqRgnMan_DS : DataStoreWrite  DataStoreName=SysI_ReqRgnMan
  SysI_ReqRgnSrv_DS : DataStoreWrite  DataStoreName=SysI_ReqRgnSrv
  SysI_SSnsrPm_DS : DataStoreWrite  DataStoreName=SysI_SSnsrPm
  SysI_SpdVeh_DS : DataStoreWrite  DataStoreName=SysI_SpdVeh
  SysI_StEngDyn_DS : DataStoreWrite  DataStoreName=SysI_StEngDyn
  SysI_StEngRun_DS : DataStoreWrite  DataStoreName=SysI_StEngRun
  SysI_StExhFlap_DS : DataStoreWrite  DataStoreName=SysI_StExhFlap
  SysI_StIgOn_DS : DataStoreWrite  DataStoreName=SysI_StIgOn
  SysI_StPmSnsrRdyToMeas_DS : DataStoreWrite  DataStoreName=SysI_StPmSnsrRdyToMeas
  SysI_StSnsrPmMeas_DS : DataStoreWrite  DataStoreName=SysI_StSnsrPmMeas
  SysI_StVehMode_DS : DataStoreWrite  DataStoreName=SysI_StVehMode
  SysI_TCoolt_DS : DataStoreWrite  DataStoreName=SysI_TCoolt
  SysI_TSnsrPmMean_DS : DataStoreWrite  DataStoreName=SysI_TSnsrPmMean
  SysI_VldSnsrAmbP_DS : DataStoreWrite  DataStoreName=SysI_VldSnsrAmbP
  SysI_VldSnsrAmbT_DS : DataStoreWrite  DataStoreName=SysI_VldSnsrAmbT
  SysI_VldSnsrPm_DS : DataStoreWrite  DataStoreName=SysI_VldSnsrPm
  wires:
  AIC_LamClcd/1 -> AIC_LamClcd_DS/1
  AIC_MfExh/1 -> AIC_MfExh_DS/1
  AIC_RateEgr/1 -> AIC_RateEgr_DS/1
  DocM_ConcNo2Ds/1 -> DocM_ConcNo2Ds_DS/1
  DocM_ConcNoDs/1 -> DocM_ConcNoDs_DS/1
  DocM_ConcOxyDocDs/1 -> DocM_ConcOxyDocDs_DS/1
  DocM_RatNo2ToNoxDocDs/1 -> DocM_RatNo2ToNoxDocDs_DS/1
  DocMgr_StHcLoffRdy/1 -> DocMgr_StHcLoffRdy_DS/1
  DocTC_EnaDocTCtl/1 -> DocTC_EnaDocTCtl_DS/1
  DocTC_TGasDocUsDmd/1 -> DocTC_TGasDocUsDmd_DS/1
  ELC_LamDmd/1 -> ELC_LamDmd_DS/1
  ESPAq_PAmb/1 -> ESPAq_PAmb_DS/1
  ESPAq_PdifDpf/1 -> ESPAq_PdifDpf_DS/1
  ESTAq_TAmb/1 -> ESTAq_TAmb_DS/1
  ESTAq_TGasDocUs/1 -> ESTAq_TGasDocUs_DS/1
  ESTAq_TGasDpfUs/1 -> ESTAq_TGasDpfUs_DS/1
  ESTAq_TGasScrDs/1 -> ESTAq_TGasScrDs_DS/1
  ESTAq_TGasScrUs/1 -> ESTAq_TGasScrUs_DS/1
  EaC_DisaDocHeatgCl/1 -> EaC_DisaDocHeatgCl_DS/1
  EaC_DisaDpfRgn/1 -> EaC_DisaDpfRgn_DS/1
  EaC_DisaSootMdlEre/1 -> EaC_DisaSootMdlEre_DS/1
  EaC_DisaSootMdlPDif/1 -> EaC_DisaSootMdlPDif_DS/1
  EaC_EnaDocProtnHeatg/1 -> EaC_EnaDocProtnHeatg_DS/1
  EaC_ReqDesox/1 -> EaC_ReqDesox_DS/1
  EaC_ReqDesoxImdty/1 -> EaC_ReqDesoxImdty_DS/1
  EaC_StOperMode/1 -> EaC_StOperMode_DS/1
  EreSAM_MconcAsh/1 -> EreSAM_MconcAsh_DS/1
  EreSAM_MconcSoot/1 -> EreSAM_MconcSoot_DS/1
  NSAq_ConcNoxScrDs/1 -> NSAq_ConcNoxScrDs_DS/1
  ScrI_MfNh3InjrRelzd/1 -> ScrI_MfNh3InjrRelzd_DS/1
  SysI_EnaDocTCtlMong/1 -> SysI_EnaDocTCtlMong_DS/1
  SysI_EnaDpfAshLoaMong/1 -> SysI_EnaDpfAshLoaMong_DS/1
  SysI_EnaDpfClgMong/1 -> SysI_EnaDpfClgMong_DS/1
  SysI_EnaDpfOvrhtMong/1 -> SysI_EnaDpfOvrhtMong_DS/1
  SysI_EnaDpfRgnMongIncmpl/1 -> SysI_EnaDpfRgnMongIncmpl_DS/1
  SysI_EnaDpfRgnMongPerd/1 -> SysI_EnaDpfRgnMongPerd_DS/1
  SysI_EnaDpfRmvlMong/1 -> SysI_EnaDpfRmvlMong_DS/1
  SysI_EnaDpfTCtlMong/1 -> SysI_EnaDpfTCtlMong_DS/1
  SysI_EnaSnsrPmMong/1 -> SysI_EnaSnsrPmMong_DS/1
  SysI_ISnsrPmSootAbsptn/1 -> SysI_ISnsrPmSootAbsptn_DS/1
  SysI_MfHcInj/1 -> SysI_MfHcInj_DS/1
  SysI_MfInj/1 -> SysI_MfInj_DS/1
  SysI_MfInjLatePost/1 -> SysI_MfInjLatePost_DS/1
  SysI_MilgDpfTot/1 -> SysI_MilgDpfTot_DS/1
  SysI_NEng/1 -> SysI_NEng_DS/1
  SysI_ReqEngStop/1 -> SysI_ReqEngStop_DS/1
  SysI_ReqRgnMan/1 -> SysI_ReqRgnMan_DS/1
  SysI_ReqRgnSrv/1 -> SysI_ReqRgnSrv_DS/1
  SysI_SSnsrPm/1 -> SysI_SSnsrPm_DS/1
  SysI_SpdVeh/1 -> SysI_SpdVeh_DS/1
  SysI_StEngDyn/1 -> SysI_StEngDyn_DS/1
  SysI_StEngRun/1 -> SysI_StEngRun_DS/1
  SysI_StExhFlap/1 -> SysI_StExhFlap_DS/1
  SysI_StIgOn/1 -> SysI_StIgOn_DS/1
  SysI_StPmSnsrRdyToMeas/1 -> SysI_StPmSnsrRdyToMeas_DS/1
  SysI_StSnsrPmMeas/1 -> SysI_StSnsrPmMeas_DS/1
  SysI_StVehMode/1 -> SysI_StVehMode_DS/1
  SysI_TCoolt/1 -> SysI_TCoolt_DS/1
  SysI_TSnsrPmMean/1 -> SysI_TSnsrPmMean_DS/1
  SysI_VldSnsrAmbP/1 -> SysI_VldSnsrAmbP_DS/1
  SysI_VldSnsrAmbT/1 -> SysI_VldSnsrAmbT_DS/1
  SysI_VldSnsrPm/1 -> SysI_VldSnsrPm_DS/1

== system DpfIntfc_Delivery/DpfIntfc/OpSys ==
  note: Help for OpSys Subsystem
  note: How to: Stimulate the AVLOpSys
  note: Use global Goto blocks
  AVLOpSys : Subsystem  mask(AVLOpSys){FixedStepSize=0.001, Types=Recurrence;Recurrence;Rising Edge;Angle based;Recurrence;Recurrence;Recurrence, Angles_Recurrences=0.02;0.02;-;180;0.02;0.02;0.02, TriggerType=Function Call;Function Call;Function Call;Function Call;Function Call;Function Call;Function Call}
      mask prompts: Types "Type"; Angles_Recurrences "Angle_Recurrence"
      mask init:
      | set_param(bdroot,'FixedStep', get_param(gcb, 'FixedStepSize'));
      settings: ModelCloseFcn=|
      | % Close open configuration window
      | if ~isempty(findobj('Tag',gcb))
      |     delete(findobj('Tag',gcb));
      | end
      settings: OpenFcn=|
      | try
      |    sl_editOpSys(gcb);
      | catch
      |    warndlg('You need AVLab to change the config of the AVLOpSys!')
      | end
      mask Display:
      | text(0.18,0.95, '{\bfAVLOpSys}', 'texmode','on')
      | text(0.18,0.85, ['Fixed step size = ' num2str(FixedStepSize)])
  Constant1 : Constant  Value=2000  SampleTime=-1
  Step1 : Step  Time=0
  Terminator : Terminator
  Terminator1 : Terminator
  tag scope: Disp_20ms=global, Input=global, OS_20ms=global, Output=global, Sti_20ms=global
  wires:
  Step1/1 -> AVLOpSys/1(Enable), AVLOpSys/3(Signal In [3])
  Constant1/1 -> AVLOpSys/2(Engine Speed)
  AVLOpSys/5(Recurrence 0.02 [5] (Fcn)) -> [OS_20ms]
  AVLOpSys/6(Recurrence 0.02 [6] (Fcn)) -> [Disp_20ms]
  AVLOpSys/2(Recurrence 0.02 [2] (Fcn)) -> [Sti_20ms]
  AVLOpSys/1(Recurrence 0.02 [1] (Fcn)) -> [Input]
  AVLOpSys/7(Recurrence 0.02 [7] (Fcn)) -> [Output]
  AVLOpSys/3(Rising Edge [3] (Fcn)) -> Terminator/1
  AVLOpSys/4(Angle based 180 [4] (Fcn)) -> Terminator1/1

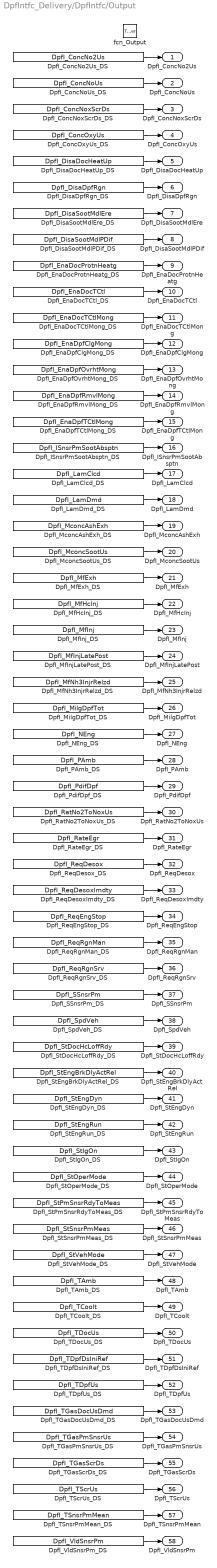
== system DpfIntfc_Delivery/DpfIntfc/Output ==
  fcn_Output : TriggerPort  TriggerType=function-call
  DpfI_ConcNo2Us_DS : DataStoreRead  DataStoreName=DpfI_ConcNo2Us
  DpfI_ConcNoUs_DS : DataStoreRead  DataStoreName=DpfI_ConcNoUs
  DpfI_ConcNoxScrDs_DS : DataStoreRead  DataStoreName=DpfI_ConcNoxScrDs
  DpfI_ConcOxyUs_DS : DataStoreRead  DataStoreName=DpfI_ConcOxyUs
  DpfI_DisaDocHeatUp_DS : DataStoreRead  DataStoreName=DpfI_DisaDocHeatUp
  DpfI_DisaDpfRgn_DS : DataStoreRead  DataStoreName=DpfI_DisaDpfRgn
  DpfI_DisaSootMdlEre_DS : DataStoreRead  DataStoreName=DpfI_DisaSootMdlEre
  DpfI_DisaSootMdlPDif_DS : DataStoreRead  DataStoreName=DpfI_DisaSootMdlPDif
  DpfI_EnaDocProtnHeatg_DS : DataStoreRead  DataStoreName=DpfI_EnaDocProtnHeatg
  DpfI_EnaDocTCtlMong_DS : DataStoreRead  DataStoreName=DpfI_EnaDocTCtlMong
  DpfI_EnaDocTCtl_DS : DataStoreRead  DataStoreName=DpfI_EnaDocTCtl
  DpfI_EnaDpfClgMong_DS : DataStoreRead  DataStoreName=DpfI_EnaDpfClgMong
  DpfI_EnaDpfOvrhtMong_DS : DataStoreRead  DataStoreName=DpfI_EnaDpfOvrhtMong
  DpfI_EnaDpfRmvlMong_DS : DataStoreRead  DataStoreName=DpfI_EnaDpfRmvlMong
  DpfI_EnaDpfTCtlMong_DS : DataStoreRead  DataStoreName=DpfI_EnaDpfTCtlMong
  DpfI_ISnsrPmSootAbsptn_DS : DataStoreRead  DataStoreName=DpfI_ISnsrPmSootAbsptn
  DpfI_LamClcd_DS : DataStoreRead  DataStoreName=DpfI_LamClcd
  DpfI_LamDmd_DS : DataStoreRead  DataStoreName=DpfI_LamDmd
  DpfI_MconcAshExh_DS : DataStoreRead  DataStoreName=DpfI_MconcAshExh
  DpfI_MconcSootUs_DS : DataStoreRead  DataStoreName=DpfI_MconcSootUs
  DpfI_MfExh_DS : DataStoreRead  DataStoreName=DpfI_MfExh
  DpfI_MfHcInj_DS : DataStoreRead  DataStoreName=DpfI_MfHcInj
  DpfI_MfInjLatePost_DS : DataStoreRead  DataStoreName=DpfI_MfInjLatePost
  DpfI_MfInj_DS : DataStoreRead  DataStoreName=DpfI_MfInj
  DpfI_MfNh3InjrRelzd_DS : DataStoreRead  DataStoreName=DpfI_MfNh3InjrRelzd
  DpfI_MilgDpfTot_DS : DataStoreRead  DataStoreName=DpfI_MilgDpfTot
  DpfI_NEng_DS : DataStoreRead  DataStoreName=DpfI_NEng
  DpfI_PAmb_DS : DataStoreRead  DataStoreName=DpfI_PAmb
  DpfI_PdifDpf_DS : DataStoreRead  DataStoreName=DpfI_PdifDpf
  DpfI_RatNo2ToNoxUs_DS : DataStoreRead  DataStoreName=DpfI_RatNo2ToNoxUs
  DpfI_RateEgr_DS : DataStoreRead  DataStoreName=DpfI_RateEgr
  DpfI_ReqDesoxImdty_DS : DataStoreRead  DataStoreName=DpfI_ReqDesoxImdty
  DpfI_ReqDesox_DS : DataStoreRead  DataStoreName=DpfI_ReqDesox
  DpfI_ReqEngStop_DS : DataStoreRead  DataStoreName=DpfI_ReqEngStop
  DpfI_ReqRgnMan_DS : DataStoreRead  DataStoreName=DpfI_ReqRgnMan
  DpfI_ReqRgnSrv_DS : DataStoreRead  DataStoreName=DpfI_ReqRgnSrv
  DpfI_SSnsrPm_DS : DataStoreRead  DataStoreName=DpfI_SSnsrPm
  DpfI_SpdVeh_DS : DataStoreRead  DataStoreName=DpfI_SpdVeh
  DpfI_StDocHcLoffRdy_DS : DataStoreRead  DataStoreName=DpfI_StDocHcLoffRdy
  DpfI_StEngBrkDlyActRel_DS : DataStoreRead  DataStoreName=DpfI_StEngBrkDlyActRel
  DpfI_StEngDyn_DS : DataStoreRead  DataStoreName=DpfI_StEngDyn
  DpfI_StEngRun_DS : DataStoreRead  DataStoreName=DpfI_StEngRun
  DpfI_StIgOn_DS : DataStoreRead  DataStoreName=DpfI_StIgOn
  DpfI_StOperMode_DS : DataStoreRead  DataStoreName=DpfI_StOperMode
  DpfI_StPmSnsrRdyToMeas_DS : DataStoreRead  DataStoreName=DpfI_StPmSnsrRdyToMeas
  DpfI_StSnsrPmMeas_DS : DataStoreRead  DataStoreName=DpfI_StSnsrPmMeas
  DpfI_StVehMode_DS : DataStoreRead  DataStoreName=DpfI_StVehMode
  DpfI_TAmb_DS : DataStoreRead  DataStoreName=DpfI_TAmb
  DpfI_TCoolt_DS : DataStoreRead  DataStoreName=DpfI_TCoolt
  DpfI_TDocUs_DS : DataStoreRead  DataStoreName=DpfI_TDocUs
  DpfI_TDpfDsIniRef_DS : DataStoreRead  DataStoreName=DpfI_TDpfDsIniRef
  DpfI_TDpfUs_DS : DataStoreRead  DataStoreName=DpfI_TDpfUs
  DpfI_TGasDocUsDmd_DS : DataStoreRead  DataStoreName=DpfI_TGasDocUsDmd
  DpfI_TGasPmSnsrUs_DS : DataStoreRead  DataStoreName=DpfI_TGasPmSnsrUs
  DpfI_TGasScrDs_DS : DataStoreRead  DataStoreName=DpfI_TGasScrDs
  DpfI_TScrUs_DS : DataStoreRead  DataStoreName=DpfI_TScrUs
  DpfI_TSnsrPmMean_DS : DataStoreRead  DataStoreName=DpfI_TSnsrPmMean
  DpfI_VldSnsrPm_DS : DataStoreRead  DataStoreName=DpfI_VldSnsrPm
  DpfI_ConcNo2Us : Outport
  DpfI_ConcNoUs : Outport  Port=2
  DpfI_ConcNoxScrDs : Outport  Port=3
  DpfI_ConcOxyUs : Outport  Port=4
  DpfI_DisaDocHeatUp : Outport  Port=5
  DpfI_DisaDpfRgn : Outport  Port=6
  DpfI_DisaSootMdlEre : Outport  Port=7
  DpfI_DisaSootMdlPDif : Outport  Port=8
  DpfI_EnaDocProtnHeatg : Outport  Port=9
  DpfI_EnaDocTCtl : Outport  Port=10
  DpfI_EnaDocTCtlMong : Outport  Port=11
  DpfI_EnaDpfClgMong : Outport  Port=12
  DpfI_EnaDpfOvrhtMong : Outport  Port=13
  DpfI_EnaDpfRmvlMong : Outport  Port=14
  DpfI_EnaDpfTCtlMong : Outport  Port=15
  DpfI_ISnsrPmSootAbsptn : Outport  Port=16
  DpfI_LamClcd : Outport  Port=17
  DpfI_LamDmd : Outport  Port=18
  DpfI_MconcAshExh : Outport  Port=19
  DpfI_MconcSootUs : Outport  Port=20
  DpfI_MfExh : Outport  Port=21
  DpfI_MfHcInj : Outport  Port=22
  DpfI_MfInj : Outport  Port=23
  DpfI_MfInjLatePost : Outport  Port=24
  DpfI_MfNh3InjrRelzd : Outport  Port=25
  DpfI_MilgDpfTot : Outport  Port=26
  DpfI_NEng : Outport  Port=27
  DpfI_PAmb : Outport  Port=28
  DpfI_PdifDpf : Outport  Port=29
  DpfI_RatNo2ToNoxUs : Outport  Port=30
  DpfI_RateEgr : Outport  Port=31
  DpfI_ReqDesox : Outport  Port=32
  DpfI_ReqDesoxImdty : Outport  Port=33
  DpfI_ReqEngStop : Outport  Port=34
  DpfI_ReqRgnMan : Outport  Port=35
  DpfI_ReqRgnSrv : Outport  Port=36
  DpfI_SSnsrPm : Outport  Port=37
  DpfI_SpdVeh : Outport  Port=38
  DpfI_StDocHcLoffRdy : Outport  Port=39
  DpfI_StEngBrkDlyActRel : Outport  Port=40
  DpfI_StEngDyn : Outport  Port=41
  DpfI_StEngRun : Outport  Port=42
  DpfI_StIgOn : Outport  Port=43
  DpfI_StOperMode : Outport  Port=44
  DpfI_StPmSnsrRdyToMeas : Outport  Port=45
  DpfI_StSnsrPmMeas : Outport  Port=46
  DpfI_StVehMode : Outport  Port=47
  DpfI_TAmb : Outport  Port=48
  DpfI_TCoolt : Outport  Port=49
  DpfI_TDocUs : Outport  Port=50
  DpfI_TDpfDsIniRef : Outport  Port=51
  DpfI_TDpfUs : Outport  Port=52
  DpfI_TGasDocUsDmd : Outport  Port=53
  DpfI_TGasPmSnsrUs : Outport  Port=54
  DpfI_TGasScrDs : Outport  Port=55
  DpfI_TScrUs : Outport  Port=56
  DpfI_TSnsrPmMean : Outport  Port=57
  DpfI_VldSnsrPm : Outport  Port=58
  wires:
  DpfI_ConcNo2Us_DS/1 -> DpfI_ConcNo2Us/1
  DpfI_ConcNoUs_DS/1 -> DpfI_ConcNoUs/1
  DpfI_ConcNoxScrDs_DS/1 -> DpfI_ConcNoxScrDs/1
  DpfI_ConcOxyUs_DS/1 -> DpfI_ConcOxyUs/1
  DpfI_DisaDocHeatUp_DS/1 -> DpfI_DisaDocHeatUp/1
  DpfI_DisaDpfRgn_DS/1 -> DpfI_DisaDpfRgn/1
  DpfI_DisaSootMdlEre_DS/1 -> DpfI_DisaSootMdlEre/1
  DpfI_DisaSootMdlPDif_DS/1 -> DpfI_DisaSootMdlPDif/1
  DpfI_EnaDocProtnHeatg_DS/1 -> DpfI_EnaDocProtnHeatg/1
  DpfI_EnaDocTCtl_DS/1 -> DpfI_EnaDocTCtl/1
  DpfI_EnaDocTCtlMong_DS/1 -> DpfI_EnaDocTCtlMong/1
  DpfI_EnaDpfClgMong_DS/1 -> DpfI_EnaDpfClgMong/1
  DpfI_EnaDpfOvrhtMong_DS/1 -> DpfI_EnaDpfOvrhtMong/1
  DpfI_EnaDpfRmvlMong_DS/1 -> DpfI_EnaDpfRmvlMong/1
  DpfI_EnaDpfTCtlMong_DS/1 -> DpfI_EnaDpfTCtlMong/1
  DpfI_ISnsrPmSootAbsptn_DS/1 -> DpfI_ISnsrPmSootAbsptn/1
  DpfI_LamClcd_DS/1 -> DpfI_LamClcd/1
  DpfI_LamDmd_DS/1 -> DpfI_LamDmd/1
  DpfI_MconcAshExh_DS/1 -> DpfI_MconcAshExh/1
  DpfI_MconcSootUs_DS/1 -> DpfI_MconcSootUs/1
  DpfI_MfExh_DS/1 -> DpfI_MfExh/1
  DpfI_MfHcInj_DS/1 -> DpfI_MfHcInj/1
  DpfI_MfInj_DS/1 -> DpfI_MfInj/1
  DpfI_MfInjLatePost_DS/1 -> DpfI_MfInjLatePost/1
  DpfI_MfNh3InjrRelzd_DS/1 -> DpfI_MfNh3InjrRelzd/1
  DpfI_MilgDpfTot_DS/1 -> DpfI_MilgDpfTot/1
  DpfI_NEng_DS/1 -> DpfI_NEng/1
  DpfI_PAmb_DS/1 -> DpfI_PAmb/1
  DpfI_PdifDpf_DS/1 -> DpfI_PdifDpf/1
  DpfI_RatNo2ToNoxUs_DS/1 -> DpfI_RatNo2ToNoxUs/1
  DpfI_RateEgr_DS/1 -> DpfI_RateEgr/1
  DpfI_ReqDesox_DS/1 -> DpfI_ReqDesox/1
  DpfI_ReqDesoxImdty_DS/1 -> DpfI_ReqDesoxImdty/1
  DpfI_ReqEngStop_DS/1 -> DpfI_ReqEngStop/1
  DpfI_ReqRgnMan_DS/1 -> DpfI_ReqRgnMan/1
  DpfI_ReqRgnSrv_DS/1 -> DpfI_ReqRgnSrv/1
  DpfI_SSnsrPm_DS/1 -> DpfI_SSnsrPm/1
  DpfI_SpdVeh_DS/1 -> DpfI_SpdVeh/1
  DpfI_StDocHcLoffRdy_DS/1 -> DpfI_StDocHcLoffRdy/1
  DpfI_StEngBrkDlyActRel_DS/1 -> DpfI_StEngBrkDlyActRel/1
  DpfI_StEngDyn_DS/1 -> DpfI_StEngDyn/1
  DpfI_StEngRun_DS/1 -> DpfI_StEngRun/1
  DpfI_StIgOn_DS/1 -> DpfI_StIgOn/1
  DpfI_StOperMode_DS/1 -> DpfI_StOperMode/1
  DpfI_StPmSnsrRdyToMeas_DS/1 -> DpfI_StPmSnsrRdyToMeas/1
  DpfI_StSnsrPmMeas_DS/1 -> DpfI_StSnsrPmMeas/1
  DpfI_StVehMode_DS/1 -> DpfI_StVehMode/1
  DpfI_TAmb_DS/1 -> DpfI_TAmb/1
  DpfI_TCoolt_DS/1 -> DpfI_TCoolt/1
  DpfI_TDocUs_DS/1 -> DpfI_TDocUs/1
  DpfI_TDpfDsIniRef_DS/1 -> DpfI_TDpfDsIniRef/1
  DpfI_TDpfUs_DS/1 -> DpfI_TDpfUs/1
  DpfI_TGasDocUsDmd_DS/1 -> DpfI_TGasDocUsDmd/1
  DpfI_TGasPmSnsrUs_DS/1 -> DpfI_TGasPmSnsrUs/1
  DpfI_TGasScrDs_DS/1 -> DpfI_TGasScrDs/1
  DpfI_TScrUs_DS/1 -> DpfI_TScrUs/1
  DpfI_TSnsrPmMean_DS/1 -> DpfI_TSnsrPmMean/1
  DpfI_VldSnsrPm_DS/1 -> DpfI_VldSnsrPm/1

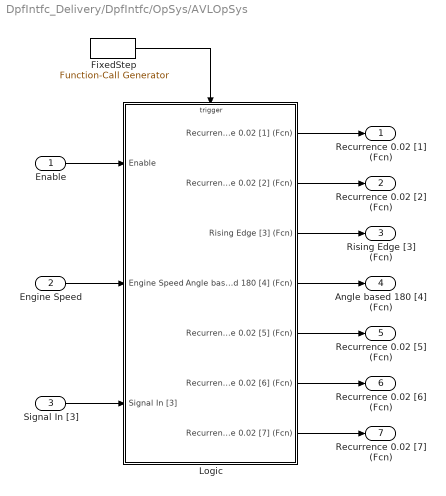
== system DpfIntfc_Delivery/DpfIntfc/OpSys/AVLOpSys ==
  Enable : Inport
  Engine Speed : Inport  Port=2
  Signal In [3] : Inport  Port=3
  FixedStep : simulink/Ports & Subsystems/Function-Call Generator  sample_time=FixedStepSize  numberOfIterations=1
      settings: AttributesFormatString=SampleTime = %<sample_time>
  Logic : Subsystem
  Recurrence 0.02 [1] (Fcn) : Outport
  Recurrence 0.02 [2] (Fcn) : Outport  Port=2
  Rising Edge [3] (Fcn) : Outport  Port=3
  Angle based 180 [4] (Fcn) : Outport  Port=4
  Recurrence 0.02 [5] (Fcn) : Outport  Port=5
  Recurrence 0.02 [6] (Fcn) : Outport  Port=6
  Recurrence 0.02 [7] (Fcn) : Outport  Port=7
  wires:
  FixedStep/1 -> Logic/Trigger
  Enable/1 -> Logic/1(Enable)
  Engine Speed/1 -> Logic/2(Engine Speed)
  Signal In [3]/1 -> Logic/3(Signal In [3])
  Logic/1(Recurrence 0.02 [1] (Fcn)) -> Recurrence 0.02 [1] (Fcn)/1
  Logic/2(Recurrence 0.02 [2] (Fcn)) -> Recurrence 0.02 [2] (Fcn)/1
  Logic/3(Rising Edge [3] (Fcn)) -> Rising Edge [3] (Fcn)/1
  Logic/4(Angle based 180 [4] (Fcn)) -> Angle based 180 [4] (Fcn)/1
  Logic/5(Recurrence 0.02 [5] (Fcn)) -> Recurrence 0.02 [5] (Fcn)/1
  Logic/6(Recurrence 0.02 [6] (Fcn)) -> Recurrence 0.02 [6] (Fcn)/1
  Logic/7(Recurrence 0.02 [7] (Fcn)) -> Recurrence 0.02 [7] (Fcn)/1

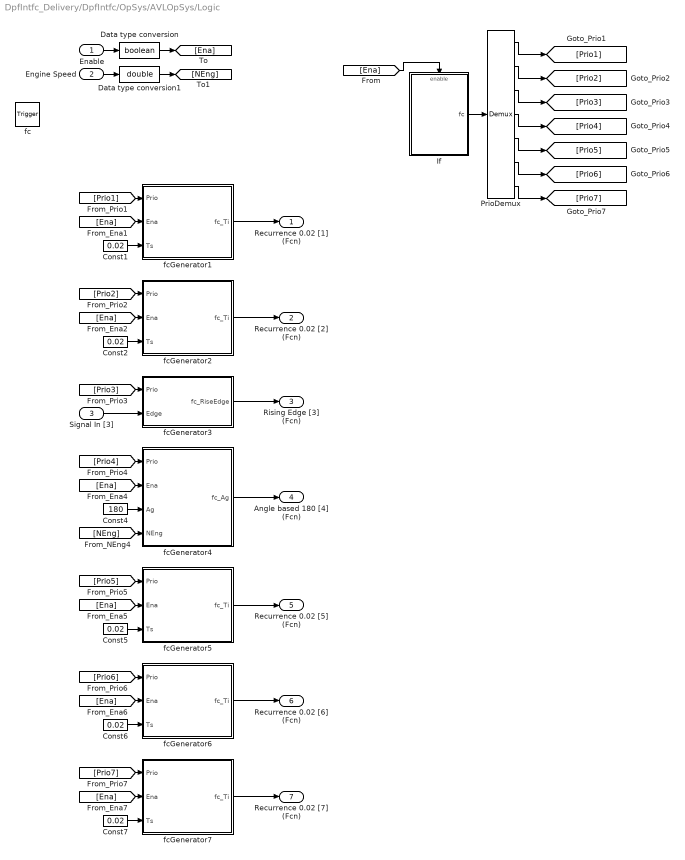
== system DpfIntfc_Delivery/DpfIntfc/OpSys/AVLOpSys/Logic ==
  Enable : Inport
  Engine Speed : Inport  Port=2
  Signal In [3] : Inport  Port=3
  fc : TriggerPort  TriggerType=function-call
  Const{1..2,5..7} (5 alike) : Constant  Value=0.02
  Const4 : Constant  Value=180
  Data type conversion : DataTypeConversion  OutDataTypeStr=boolean  SaturateOnIntegerOverflow=on  RndMeth=Zero
  Data type conversion1 : DataTypeConversion  OutDataTypeStr=double  SaturateOnIntegerOverflow=on  RndMeth=Zero
  If : Subsystem  TreatAsAtomicUnit=on
  PrioDemux : Demux  Outputs=7
  fcGenerator1 : Subsystem  Tag=fcGenerator
  fcGenerator2 : Subsystem  Tag=fcGenerator
  fcGenerator3 : Subsystem  Tag=fcGenerator
  fcGenerator4 : Subsystem  Tag=fcGenerator
  fcGenerator5 : Subsystem  Tag=fcGenerator
  fcGenerator6 : Subsystem  Tag=fcGenerator
  fcGenerator7 : Subsystem  Tag=fcGenerator
  Recurrence 0.02 [1] (Fcn) : Outport
  Recurrence 0.02 [2] (Fcn) : Outport  Port=2
  Rising Edge [3] (Fcn) : Outport  Port=3
  Angle based 180 [4] (Fcn) : Outport  Port=4
  Recurrence 0.02 [5] (Fcn) : Outport  Port=5
  Recurrence 0.02 [6] (Fcn) : Outport  Port=6
  Recurrence 0.02 [7] (Fcn) : Outport  Port=7
  wires:
  If/1(fc) -> PrioDemux/1
  [Ena] -> If/Enable
  Data type conversion1/1 -> [NEng]
  Engine Speed/1 -> Data type conversion1/1
  Data type conversion/1 -> [Ena]
  Enable/1 -> Data type conversion/1
  PrioDemux/1 -> [Prio1]
  PrioDemux/2 -> [Prio2]
  PrioDemux/3 -> [Prio3]
  PrioDemux/4 -> [Prio4]
  PrioDemux/5 -> [Prio5]
  PrioDemux/6 -> [Prio6]
  PrioDemux/7 -> [Prio7]
  [Prio1] -> fcGenerator1/1(Prio)
  [Ena] -> fcGenerator1/2(Ena)
  Const1/1 -> fcGenerator1/3(Ts)
  fcGenerator1/1(fc_Ti) -> Recurrence 0.02 [1] (Fcn)/1
  [Prio2] -> fcGenerator2/1(Prio)
  [Ena] -> fcGenerator2/2(Ena)
  Const2/1 -> fcGenerator2/3(Ts)
  fcGenerator2/1(fc_Ti) -> Recurrence 0.02 [2] (Fcn)/1
  [Prio3] -> fcGenerator3/1(Prio)
  Signal In [3]/1 -> fcGenerator3/2(Edge)
  fcGenerator3/1(fc_RiseEdge) -> Rising Edge [3] (Fcn)/1
  [Prio4] -> fcGenerator4/1(Prio)
  [Ena] -> fcGenerator4/2(Ena)
  Const4/1 -> fcGenerator4/3(Ag)
  [NEng] -> fcGenerator4/4(NEng)
  fcGenerator4/1(fc_Ag) -> Angle based 180 [4] (Fcn)/1
  [Prio5] -> fcGenerator5/1(Prio)
  [Ena] -> fcGenerator5/2(Ena)
  Const5/1 -> fcGenerator5/3(Ts)
  fcGenerator5/1(fc_Ti) -> Recurrence 0.02 [5] (Fcn)/1
  [Prio6] -> fcGenerator6/1(Prio)
  [Ena] -> fcGenerator6/2(Ena)
  Const6/1 -> fcGenerator6/3(Ts)
  fcGenerator6/1(fc_Ti) -> Recurrence 0.02 [6] (Fcn)/1
  [Prio7] -> fcGenerator7/1(Prio)
  [Ena] -> fcGenerator7/2(Ena)
  Const7/1 -> fcGenerator7/3(Ts)
  fcGenerator7/1(fc_Ti) -> Recurrence 0.02 [7] (Fcn)/1

== system DpfIntfc_Delivery/DpfIntfc/OpSys/AVLOpSys/Logic/If ==
  Enable : EnablePort
  Function-Call Generator : simulink/Ports & Subsystems/Function-Call Generator  sample_time=-1  numberOfIterations=1
  fc : Outport
  wires:
  Function-Call Generator/1 -> fc/1

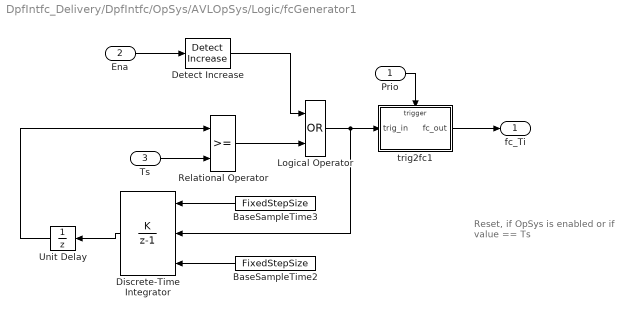
== system DpfIntfc_Delivery/DpfIntfc/OpSys/AVLOpSys/Logic/fcGenerator1 ==
  note: Reset, if OpSys is enabled or if value == Ts
  Prio : Inport
  Ena : Inport  Port=2
  Ts : Inport  Port=3
  BaseSampleTime2 : Constant  Value=FixedStepSize
  BaseSampleTime3 : Constant  Value=FixedStepSize
  Detect Increase : simulink/Logic and Bit Operations/Detect Increase  vinit=0.0  InputProcessing=Inherited  OutDataTypeStr=uint8
  Discrete-Time Integrator : DiscreteIntegrator  IntegratorMethod=Accumulation: Forward Euler  ExternalReset=rising  InitialConditionSource=external  SampleTime=-1  ICPrevOutput=DiscIntNeverNeededParam  ICPrevScaledInput=DiscIntNeverNeededParam
  Logical Operator : Logic  Operator=OR  AllPortsSameDT=off  OutDataTypeStr=boolean
  Relational Operator : RelationalOperator  OutDataTypeStr=boolean
  Unit Delay : UnitDelay  SampleTime=-1
  trig2fc1 : Subsystem
  fc_Ti : Outport
  wires:
  Unit Delay/1 -> Relational Operator/1
  Detect Increase/1 -> Logical Operator/1
  Logical Operator/1 -> Discrete-Time Integrator/2, trig2fc1/1(trig_in)
  Relational Operator/1 -> Logical Operator/2
  Ena/1 -> Detect Increase/1
  Discrete-Time Integrator/1 -> Unit Delay/1
  BaseSampleTime3/1 -> Discrete-Time Integrator/1
  BaseSampleTime2/1 -> Discrete-Time Integrator/3
  trig2fc1/1(fc_out) -> fc_Ti/1
  Prio/1 -> trig2fc1/Trigger
  Ts/1 -> Relational Operator/2
